simulink model "EnvironmentalControlSystem"  (R2018b)
settings: Solver=FixedStepAuto  StartTime=0.0  StopTime=500  FixedStep=0.01  RelTol=1e-3
values from neighbouring files (symbols this model uses):
  dt = 0.01    [run_sim.m]    (also in sys_id_pipeline.m = mean(diff(Time_vec_full)))
  K31 = Result31.K_slope    [sys_id_pipeline.m]
  K32 = Result32.K_slope    [sys_id_pipeline.m]
  P_ref = GlobalParams.P_ref    [sys_id_pipeline.m]
  Patm = GlobalParams.Patm    [sys_id_pipeline.m]
  R_gas = GlobalParams.R    [sys_id_pipeline.m]
  T_ref = GlobalParams.T_ref    [sys_id_pipeline.m]
  Tau31 = 5    [sys_id_pipeline.m]
  Tau32 = 5    [sys_id_pipeline.m]
  Tp31 = Result31.Tp    [sys_id_pipeline.m]
  Tp32 = Result32.Tp    [sys_id_pipeline.m]
  V_vol = pi * (0.05)^2 * 5    (= 0.0392699081699)    [run_sim.m]
  X31_den = sys_X31.Denominator    [sys_id_value.m]
  X31_num = sys_X31.Numerator    [sys_id_value.m]
  X32_den = sys_X32.Denominator    [sys_id_value.m]
  X32_num = sys_X32.Numerator    [sys_id_value.m]
libraries: simulink x14
(part 1 of 3)
settings Model: Creator=ZhaoJiance  LastModifiedBy=ZhaoJiance

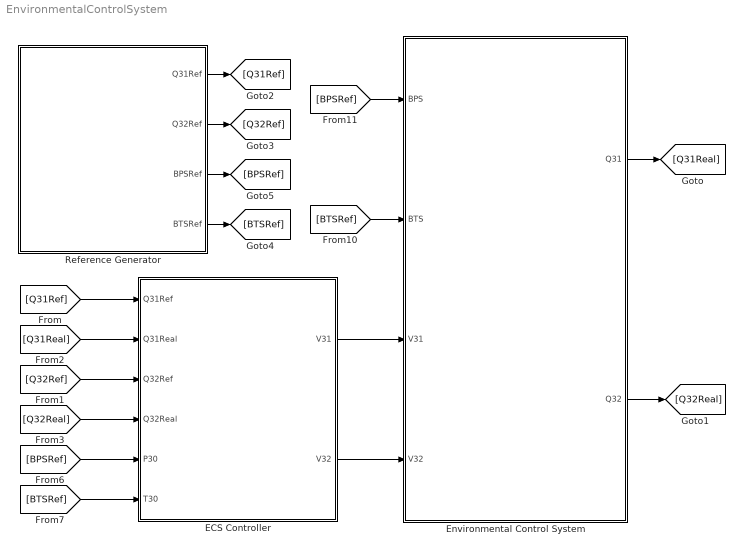
== system EnvironmentalControlSystem ==
  ECS Controller : Subsystem  VariantControlMode=Label  Variant=on  VariantControl=Variant1  LabelModeActiveChoice=Smith_MPC_Controller
  Environmental Control System : Subsystem
  Reference Generator : Subsystem
  wires:
  Reference Generator/4(BTSRef) -> [BTSRef]
  Reference Generator/2(Q32Ref) -> [Q32Ref]
  Reference Generator/3(BPSRef) -> [BPSRef]
  [BPSRef] -> Environmental Control System/1(BPS)
  [Q31Real] -> ECS Controller/2("Q31Real ")
  [BTSRef] -> Environmental Control System/2(BTS)
  [BTSRef] -> ECS Controller/6("T30 ")
  [Q32Ref] -> ECS Controller/3("Q32Ref ")
  [BPSRef] -> ECS Controller/5("P30 ")
  [Q31Ref] -> ECS Controller/1("Q31Ref ")
  Reference Generator/1(Q31Ref) -> [Q31Ref]
  [Q32Real] -> ECS Controller/4("Q32Real ")
  ECS Controller/1(" V31") -> Environmental Control System/3(V31)
  Environmental Control System/1(Q31) -> [Q31Real]
  ECS Controller/2(" V32") -> Environmental Control System/4(V32)
  Environmental Control System/2(Q32) -> [Q32Real]

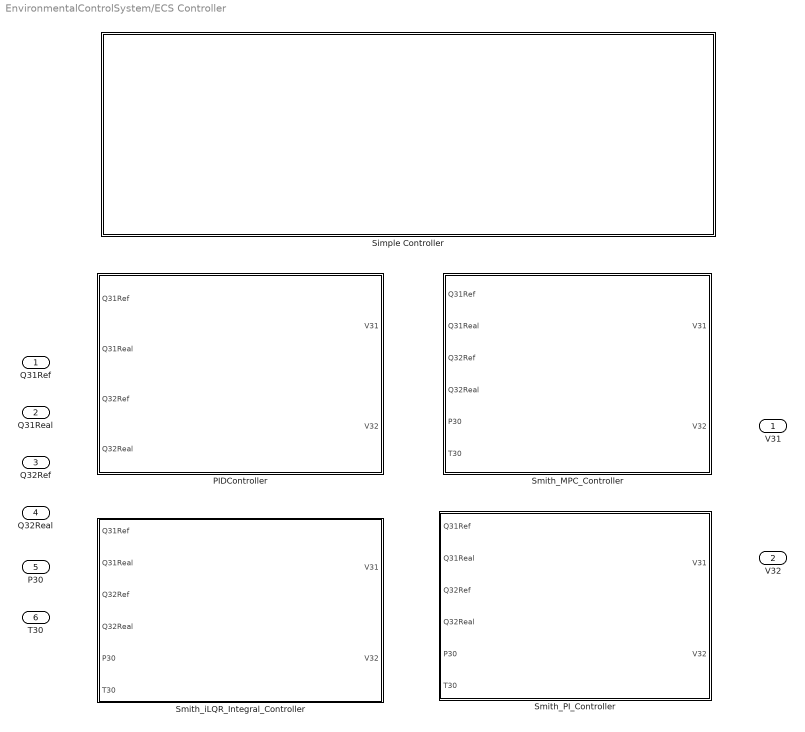
== system EnvironmentalControlSystem/ECS Controller ==
  "Q31Ref " : Inport
  "Q31Real " : Inport  Port=2
  "Q32Ref " : Inport  Port=3
  "Q32Real " : Inport  Port=4
  "P30 " : Inport  Port=5
  "T30 " : Inport  Port=6
  PIDController : Subsystem  VariantControl=PID
  Simple Controller : Subsystem  VariantControl=Variant
  Smith_MPC_Controller : Subsystem  VariantControl=Smith_MPC_Controller
  Smith_PI_Controller : Subsystem  VariantControl=Smith_PI_Controller
  Smith_iLQR_Integral_Controller : Subsystem  VariantControl=Smith_iLQR_Integral_Controller
  " V31" : Outport
  " V32" : Outport  Port=2

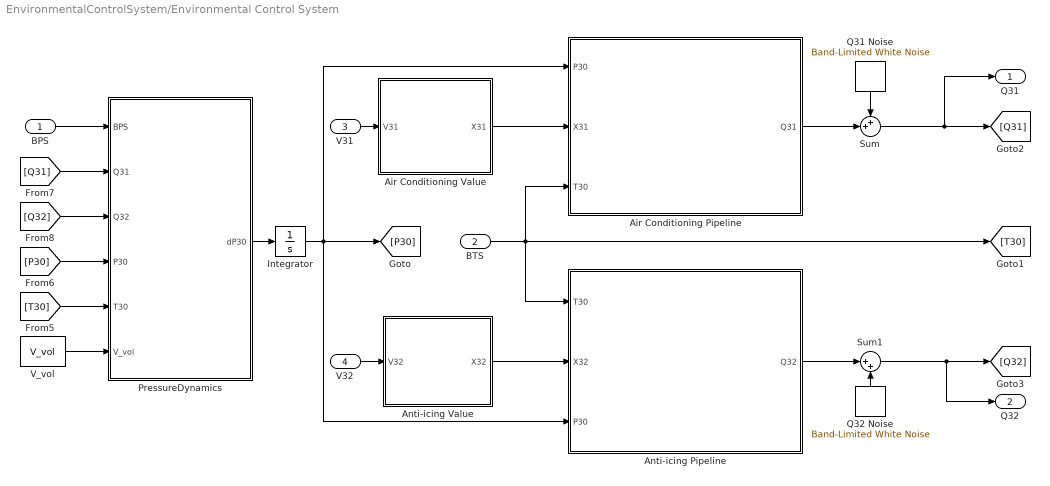
== system EnvironmentalControlSystem/Environmental Control System ==
  BPS : Inport
  BTS : Inport  Port=2
  V31 : Inport  Port=3
  V32 : Inport  Port=4
  Air Conditioning Pipeline : Subsystem
  Air Conditioning Value : Subsystem
  "Anti-icing Pipeline " : Subsystem
  Anti-icing Value : Subsystem
  Integrator : Integrator
  PressureDynamics : MATLAB Function  TreatAsAtomicUnit=on
  Q31 Noise : simulink/Sources/Band-Limited White Noise  Cov=Knoise  Ts=0.01  seed=[23341]
  Q32 Noise : simulink/Sources/Band-Limited White Noise  Cov=Knoise  Ts=0.01  seed=[23341]
  Sum : Sum  Inputs=++|
  Sum1 : Sum  Inputs=|++
  V_vol : Constant  Value=V_vol
  Q31 : Outport
  Q32 : Outport  Port=2
  wires:
  Air Conditioning Value/1(X31) -> Air Conditioning Pipeline/2(X31)
  BPS/1 -> PressureDynamics/1(BPS)
  Integrator/1 -> "Anti-icing Pipeline "/3(P30), [P30], Air Conditioning Pipeline/1(P30)
  Anti-icing Value/1(X32) -> "Anti-icing Pipeline "/2(X32)
  V31/1 -> Air Conditioning Value/1(V31)
  PressureDynamics/1(dP30) -> Integrator/1
  [Q32] -> PressureDynamics/3(Q32)
  [Q31] -> PressureDynamics/2(Q31)
  V_vol/1 -> PressureDynamics/6(V_vol)
  [P30] -> PressureDynamics/4(P30)
  [T30] -> PressureDynamics/5(T30)
  BTS/1 -> Air Conditioning Pipeline/3(T30), [T30], "Anti-icing Pipeline "/1(T30)
  Sum/1 -> [Q31], Q31/1
  Sum1/1 -> Q32/1, [Q32]
  Q32 Noise/1 -> Sum1/2
  "Anti-icing Pipeline "/1(Q32) -> Sum1/1
  Air Conditioning Pipeline/1(Q31) -> Sum/2
  Q31 Noise/1 -> Sum/1
  V32/1 -> Anti-icing Value/1(V32)

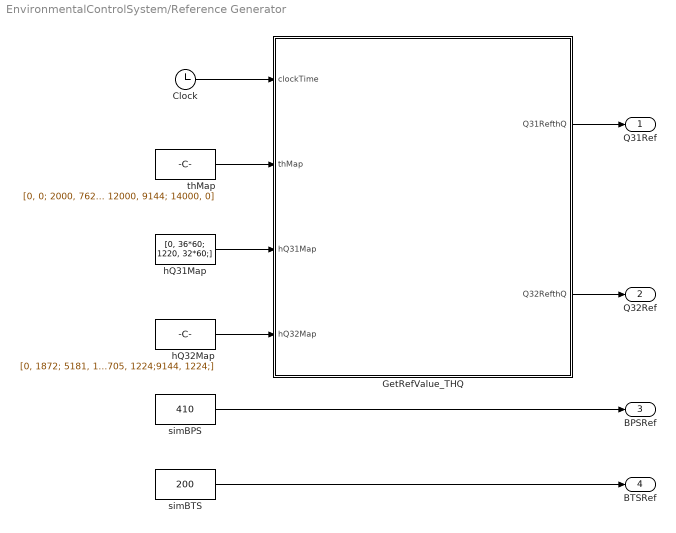
== system EnvironmentalControlSystem/Reference Generator ==
  Clock : Clock
  GetRefValue_THQ : MATLAB Function  TreatAsAtomicUnit=on
  hQ31Map : Constant  Value=[0, 36*60; 1220, 32*60;]
  hQ32Map : Constant  Value=[0, 1872; 5181, 1872; 6705, 1224;9144, 1224;]
  simBPS : Constant  Value=410
  simBTS : Constant  Value=200
  thMap : Constant  Value=[0, 0; 2000, 7620; 4000, 7620;6000, 12192; 8000, 12192; 10000, 9144; 12000, 9144; 14000, 0]
  Q31Ref : Outport
  Q32Ref : Outport  Port=2
  BPSRef : Outport  Port=3
  BTSRef : Outport  Port=4
  wires:
  Clock/1 -> GetRefValue_THQ/1(clockTime)
  thMap/1 -> GetRefValue_THQ/2(thMap)
  hQ31Map/1 -> GetRefValue_THQ/3(hQ31Map)
  hQ32Map/1 -> GetRefValue_THQ/4(hQ32Map)
  simBTS/1 -> BTSRef/1
  simBPS/1 -> BPSRef/1
  GetRefValue_THQ/1(Q31RefthQ) -> Q31Ref/1
  GetRefValue_THQ/2(Q32RefthQ) -> Q32Ref/1

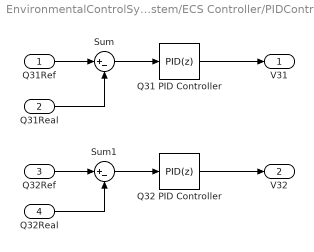
== system EnvironmentalControlSystem/ECS Controller/PIDController ==
  Q31Ref : Inport
  Q31Real : Inport  Port=2
  Q32Ref : Inport  Port=3
  Q32Real : Inport  Port=4
  Q31 PID Controller : simulink/Continuous/PID Controller  Controller=PID  Form=Parallel  TimeDomain=Discrete-time  SampleTime=-1  IntegratorMethod=Forward Euler  FilterMethod=Forward Euler  ControllerParametersSource=internal  P=0.0332634866006577  I=0.00162963841502539  D=0.0693776015925971  UseFilter=on  N=0.140831158638555  TunerSelectOption=Transfer Function Based (PID Tuner App)  InitialConditionSource=internal  InitialConditionForIntegrator=0  InitialConditionForFilter=0  DifferentiatorICPrevScaledInput=0  ExternalReset=none  TrackingMode=off  Kt=1  LimitOutput=off  UpperSaturationLimit=inf  LowerSaturationLimit=-inf  LinearizeAsGain=on  AntiWindupMode=none  Kb=1  POutMin=[]  POutMax=[]  IOutMin=[]  IOutMax=[]  DOutMin=[]  DOutMax=[]  NOutMin=[]  NOutMax=[]  SumOutMin=[]  SumOutMax=[]  SaturationOutMin=[]  SaturationOutMax=[]  PParamMin=[]  PParamMax=[]  IParamMin=[]  IParamMax=[]  DParamMin=[]  DParamMax=[]  NParamMin=[]  NParamMax=[]  KbParamMin=[]  KbParamMax=[]  KtParamMin=[]  KtParamMax=[]  KbOutMin=[]  KbOutMax=[]  KtOutMin=[]  KtOutMax=[]  IntegratorOutMin=[]  IntegratorOutMax=[]  FilterOutMin=[]  FilterOutMax=[]  SumI1OutMin=[]  SumI1OutMax=[]  SumI2OutMin=[]  SumI2OutMax=[]  SumI3OutMin=[]  SumI3OutMax=[]  SumI4OutMin=[]  SumI4OutMax=[]  SumDOutMin=[]  SumDOutMax=[]  DifferentiatorOutMin=[]  DifferentiatorOutMax=[]  FilterDiffOutCoefMin=[]  FilterDiffOutCoefMax=[]  ReciprocalOutMin=[]  ReciprocalOutMax=[]  SumDenOutMin=[]  SumDenOutMax=[]  SumNumOutMin=[]  SumNumOutMax=[]  DivideOutMin=[]  DivideOutMax=[]  IntegratorContinuousStateAttributes=''  IntegratorStateMustResolveToSignalObject=off  IntegratorRTWStateStorageClass=Auto  FilterContinuousStateAttributes=''  FilterStateMustResolveToSignalObject=off  FilterRTWStateStorageClass=Auto  ParallelPVariant=InternalParameters  IdealPVariant=Disabled  IVariant=InternalParameters  DVariant=InternalParameters  IntegratorVariant=Discrete  SatVariant=Disabled  AWVariant=Passthrough  PCopyVariant=Disabled  TRVariant=Disabled  FdbkBlocksVariant=Forward  IdealPFdbkVariant=Disabled  SatFdbkVariant=Disabled  DerivativeFilterVariant=ForwardEulerFilter  NVariant=InternalParameters  NCopyVariant=Disabled  FilterICVariant=InternalICsFilter  IntegratorICVariant=InternalICs  ExternalResetVariant=Disabled  TRSumVariant=Passthrough  SumFdbkVariant=Disabled  SumVariant=Sum_PID
  Q32 PID Controller : simulink/Continuous/PID Controller  Controller=PID  Form=Parallel  TimeDomain=Discrete-time  SampleTime=-1  IntegratorMethod=Forward Euler  FilterMethod=Forward Euler  ControllerParametersSource=internal  P=0.0550164924963942  I=0.00248684748202474  D=0.0884119468512251  UseFilter=on  N=14.1148734165854  TunerSelectOption=Transfer Function Based (PID Tuner App)  InitialConditionSource=internal  InitialConditionForIntegrator=0  InitialConditionForFilter=0  DifferentiatorICPrevScaledInput=0  ExternalReset=none  TrackingMode=off  Kt=1  LimitOutput=off  UpperSaturationLimit=inf  LowerSaturationLimit=-inf  LinearizeAsGain=on  AntiWindupMode=none  Kb=1  POutMin=[]  POutMax=[]  IOutMin=[]  IOutMax=[]  DOutMin=[]  DOutMax=[]  NOutMin=[]  NOutMax=[]  SumOutMin=[]  SumOutMax=[]  SaturationOutMin=[]  SaturationOutMax=[]  PParamMin=[]  PParamMax=[]  IParamMin=[]  IParamMax=[]  DParamMin=[]  DParamMax=[]  NParamMin=[]  NParamMax=[]  KbParamMin=[]  KbParamMax=[]  KtParamMin=[]  KtParamMax=[]  KbOutMin=[]  KbOutMax=[]  KtOutMin=[]  KtOutMax=[]  IntegratorOutMin=[]  IntegratorOutMax=[]  FilterOutMin=[]  FilterOutMax=[]  SumI1OutMin=[]  SumI1OutMax=[]  SumI2OutMin=[]  SumI2OutMax=[]  SumI3OutMin=[]  SumI3OutMax=[]  SumI4OutMin=[]  SumI4OutMax=[]  SumDOutMin=[]  SumDOutMax=[]  DifferentiatorOutMin=[]  DifferentiatorOutMax=[]  FilterDiffOutCoefMin=[]  FilterDiffOutCoefMax=[]  ReciprocalOutMin=[]  ReciprocalOutMax=[]  SumDenOutMin=[]  SumDenOutMax=[]  SumNumOutMin=[]  SumNumOutMax=[]  DivideOutMin=[]  DivideOutMax=[]  IntegratorContinuousStateAttributes=''  IntegratorStateMustResolveToSignalObject=off  IntegratorRTWStateStorageClass=Auto  FilterContinuousStateAttributes=''  FilterStateMustResolveToSignalObject=off  FilterRTWStateStorageClass=Auto  ParallelPVariant=InternalParameters  IdealPVariant=Disabled  IVariant=InternalParameters  DVariant=InternalParameters  IntegratorVariant=Discrete  SatVariant=Disabled  AWVariant=Passthrough  PCopyVariant=Disabled  TRVariant=Disabled  FdbkBlocksVariant=Forward  IdealPFdbkVariant=Disabled  SatFdbkVariant=Disabled  DerivativeFilterVariant=ForwardEulerFilter  NVariant=InternalParameters  NCopyVariant=Disabled  FilterICVariant=InternalICsFilter  IntegratorICVariant=InternalICs  ExternalResetVariant=Disabled  TRSumVariant=Passthrough  SumFdbkVariant=Disabled  SumVariant=Sum_PID
  Sum : Sum  Inputs=|+-
  Sum1 : Sum  Inputs=|+-
  V31 : Outport
  V32 : Outport  Port=2
  wires:
  Q31Ref/1 -> Sum/1
  Sum/1 -> Q31 PID Controller/1
  Q32Real/1 -> Sum1/2
  Q32Ref/1 -> Sum1/1
  Q31Real/1 -> Sum/2
  Q31 PID Controller/1 -> V31/1
  Q32 PID Controller/1 -> V32/1
  Sum1/1 -> Q32 PID Controller/1

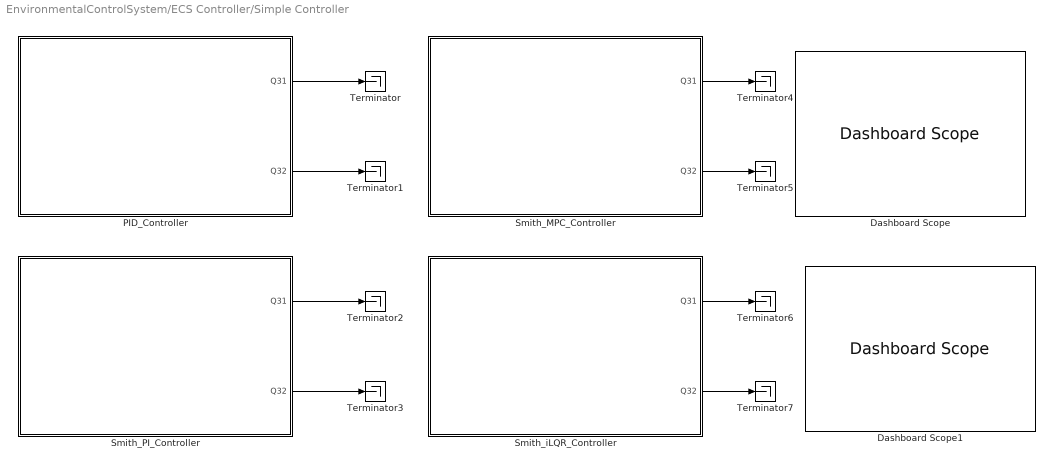
== system EnvironmentalControlSystem/ECS Controller/Simple Controller ==
  Dashboard Scope : DashboardScope  WebBlockId=462
  Dashboard Scope1 : DashboardScope  WebBlockId=463
  PID_Controller : Subsystem
  Smith_MPC_Controller : Subsystem
  Smith_PI_Controller : Subsystem
  Smith_iLQR_Controller : Subsystem
  Terminator{,1..7} (8 alike) : Terminator
  wires:
  Smith_iLQR_Controller/1(Q31) -> Terminator6/1
  PID_Controller/1(Q31) -> Terminator/1
  Smith_iLQR_Controller/2(Q32) -> Terminator7/1
  Smith_PI_Controller/2(Q32) -> Terminator3/1
  Smith_MPC_Controller/1(Q31) -> Terminator4/1
  PID_Controller/2(Q32) -> Terminator1/1
  Smith_MPC_Controller/2(Q32) -> Terminator5/1
  Smith_PI_Controller/1(Q31) -> Terminator2/1

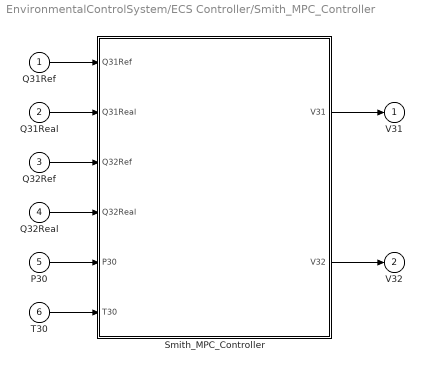
== system EnvironmentalControlSystem/ECS Controller/Smith_MPC_Controller ==
  "Q31Ref " : Inport
  "Q31Real " : Inport  Port=2
  "Q32Ref " : Inport  Port=3
  "Q32Real " : Inport  Port=4
  "P30 " : Inport  Port=5
  "T30 " : Inport  Port=6
  Smith_MPC_Controller : MATLAB Function  TreatAsAtomicUnit=on
  " V31" : Outport
  " V32" : Outport  Port=2
  wires:
  "Q31Ref "/1 -> Smith_MPC_Controller/1(Q31Ref)
  "Q31Real "/1 -> Smith_MPC_Controller/2(Q31Real)
  "T30 "/1 -> Smith_MPC_Controller/6(T30)
  "P30 "/1 -> Smith_MPC_Controller/5(P30)
  "Q32Real "/1 -> Smith_MPC_Controller/4(Q32Real)
  "Q32Ref "/1 -> Smith_MPC_Controller/3(Q32Ref)
  Smith_MPC_Controller/2(V32) -> " V32"/1
  Smith_MPC_Controller/1(V31) -> " V31"/1

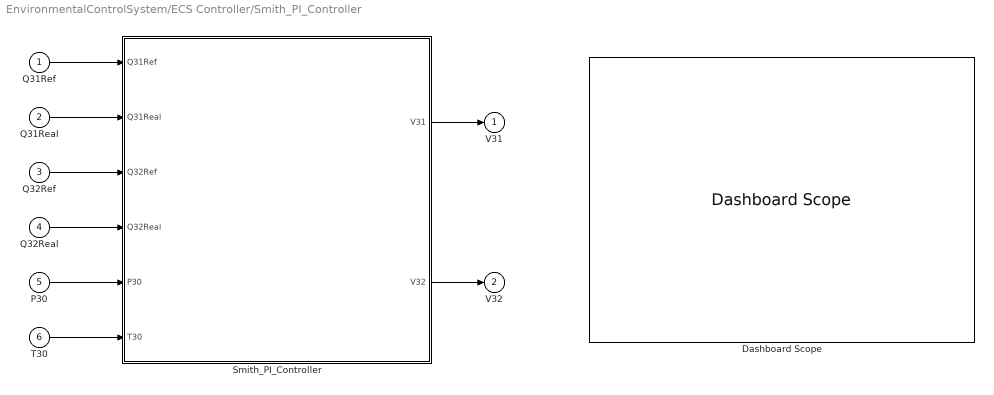
== system EnvironmentalControlSystem/ECS Controller/Smith_PI_Controller ==
  "Q31Ref " : Inport
  "Q31Real " : Inport  Port=2
  "Q32Ref " : Inport  Port=3
  "Q32Real " : Inport  Port=4
  "P30 " : Inport  Port=5
  "T30 " : Inport  Port=6
  Dashboard Scope : DashboardScope  WebBlockId=445
  Smith_PI_Controller : MATLAB Function  TreatAsAtomicUnit=on
  " V31" : Outport
  " V32" : Outport  Port=2
  wires:
  Smith_PI_Controller/1(V31) -> " V31"/1
  Smith_PI_Controller/2(V32) -> " V32"/1
  "Q31Ref "/1 -> Smith_PI_Controller/1(Q31Ref)
  "Q31Real "/1 -> Smith_PI_Controller/2(Q31Real)
  "Q32Ref "/1 -> Smith_PI_Controller/3(Q32Ref)
  "Q32Real "/1 -> Smith_PI_Controller/4(Q32Real)
  "P30 "/1 -> Smith_PI_Controller/5(P30)
  "T30 "/1 -> Smith_PI_Controller/6(T30)

== system EnvironmentalControlSystem/ECS Controller/Smith_iLQR_Integral_Controller ==
  "Q31Ref " : Inport
  "Q31Real " : Inport  Port=2
  "Q32Ref " : Inport  Port=3
  "Q32Real " : Inport  Port=4
  "P30 " : Inport  Port=5
  "T30 " : Inport  Port=6
  Smith_iLQR_Integral_Controller : MATLAB Function  TreatAsAtomicUnit=on
  " V31" : Outport
  " V32" : Outport  Port=2
  wires:
  Smith_iLQR_Integral_Controller/1(V31) -> " V31"/1
  Smith_iLQR_Integral_Controller/2(V32) -> " V32"/1
  "Q31Real "/1 -> Smith_iLQR_Integral_Controller/2(Q31Real)
  "Q31Ref "/1 -> Smith_iLQR_Integral_Controller/1(Q31Ref)
  "Q32Ref "/1 -> Smith_iLQR_Integral_Controller/3(Q32Ref)
  "Q32Real "/1 -> Smith_iLQR_Integral_Controller/4(Q32Real)
  "P30 "/1 -> Smith_iLQR_Integral_Controller/5(P30)
  "T30 "/1 -> Smith_iLQR_Integral_Controller/6(T30)

== system EnvironmentalControlSystem/Environmental Control System/Air Conditioning Pipeline ==
  P30 : Inport
  X31 : Inport  Port=2
  T30 : Inport  Port=3
  MATLAB Function : MATLAB Function  TreatAsAtomicUnit=on
  Saturation : Saturate  UpperLimit=inf  LowerLimit=0
  Transfer Fcn : TransferFcn  Denominator=[Tp31 1]
  Transport Delay : TransportDelay  DelayTime=Tau31
  Q31 : Outport
  wires:
  Transfer Fcn/1 -> Transport Delay/1
  X31/1 -> MATLAB Function/1(X)
  MATLAB Function/1(Q_static) -> Transfer Fcn/1
  T30/1 -> MATLAB Function/3(T30)
  P30/1 -> MATLAB Function/2(P30)
  Transport Delay/1 -> Saturation/1
  Saturation/1 -> Q31/1

== system EnvironmentalControlSystem/Environmental Control System/Air Conditioning Value ==
  V31 : Inport
  V31Saturation : Saturate  UpperLimit=100  LowerLimit=0
  X31 Saturation : Saturate  UpperLimit=100  LowerLimit=0
  X31 Value System : TransferFcn  Numerator=X31_num  Denominator=X31_den
  X31Deadband : MATLAB Function  TreatAsAtomicUnit=on  SystemSampleTime=0.01
  X31 : Outport
  wires:
  X31Deadband/1(u_eff) -> X31 Value System/1
  X31 Saturation/1 -> X31/1, X31Deadband/1(curPos)
  X31 Value System/1 -> X31 Saturation/1
  V31/1 -> V31Saturation/1
  V31Saturation/1 -> X31Deadband/2(cmdPos)

== system EnvironmentalControlSystem/Environmental Control System/Anti-icing Pipeline  ==
  T30 : Inport
  X32 : Inport  Port=2
  P30 : Inport  Port=3
  MATLAB Function : MATLAB Function  TreatAsAtomicUnit=on
  Saturation : Saturate  UpperLimit=inf  LowerLimit=0
  Transfer Fcn : TransferFcn  Denominator=[Tp32 1]
  Transport Delay : TransportDelay  DelayTime=Tau32
  Q32 : Outport
  wires:
  P30/1 -> MATLAB Function/2(P30)
  MATLAB Function/1(Q_static) -> Transfer Fcn/1
  Transfer Fcn/1 -> Transport Delay/1
  T30/1 -> MATLAB Function/3(T30)
  Transport Delay/1 -> Saturation/1
  X32/1 -> MATLAB Function/1(X)
  Saturation/1 -> Q32/1

== system EnvironmentalControlSystem/Environmental Control System/Anti-icing Value ==
  V32 : Inport
  V32 Saturation : Saturate  UpperLimit=100  LowerLimit=0
  X32 Saturation : Saturate  UpperLimit=100  LowerLimit=0
  X32 Value System : TransferFcn  Numerator=X32_num  Denominator=X32_den
  X32Deadband : MATLAB Function  TreatAsAtomicUnit=on  SystemSampleTime=0.01
  X32 : Outport
  wires:
  V32/1 -> V32 Saturation/1
  X32Deadband/1(u_eff) -> X32 Value System/1
  X32 Saturation/1 -> X32/1, X32Deadband/1(curPos)
  X32 Value System/1 -> X32 Saturation/1
  V32 Saturation/1 -> X32Deadband/2(cmdPos)

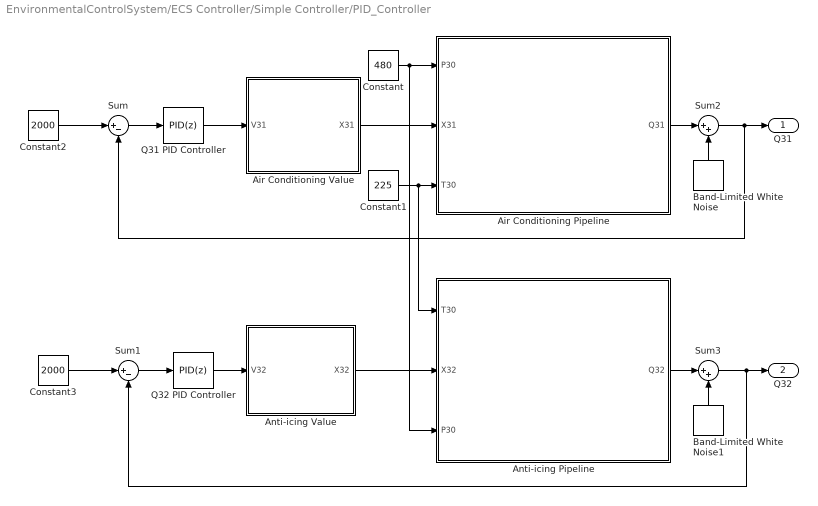
== system EnvironmentalControlSystem/ECS Controller/Simple Controller/PID_Controller ==
  Air Conditioning Pipeline : Subsystem
  Air Conditioning Value : Subsystem
  "Anti-icing Pipeline " : Subsystem
  Anti-icing Value : Subsystem
  Band-Limited White Noise : simulink/Sources/Band-Limited White Noise  Cov=Knoise  Ts=0.1  seed=[23341]
  Band-Limited White Noise1 : simulink/Sources/Band-Limited White Noise  Cov=Knoise  Ts=0.1  seed=[23341]
  Constant : Constant  Value=480
  Constant1 : Constant  Value=225
  Constant2 : Constant  Value=2000
  Constant3 : Constant  Value=2000
  Q31 PID Controller : simulink/Continuous/PID Controller  Controller=PID  Form=Parallel  TimeDomain=Discrete-time  SampleTime=-1  IntegratorMethod=Forward Euler  FilterMethod=Forward Euler  ControllerParametersSource=internal  P=0.0332634866006577  I=0.00162963841502539  D=0.0693776015925971  UseFilter=on  N=0.140831158638555  TunerSelectOption=Transfer Function Based (PID Tuner App)  InitialConditionSource=internal  InitialConditionForIntegrator=0  InitialConditionForFilter=0  DifferentiatorICPrevScaledInput=0  ExternalReset=none  TrackingMode=off  Kt=1  LimitOutput=off  UpperSaturationLimit=inf  LowerSaturationLimit=-inf  LinearizeAsGain=on  AntiWindupMode=none  Kb=1  POutMin=[]  POutMax=[]  IOutMin=[]  IOutMax=[]  DOutMin=[]  DOutMax=[]  NOutMin=[]  NOutMax=[]  SumOutMin=[]  SumOutMax=[]  SaturationOutMin=[]  SaturationOutMax=[]  PParamMin=[]  PParamMax=[]  IParamMin=[]  IParamMax=[]  DParamMin=[]  DParamMax=[]  NParamMin=[]  NParamMax=[]  KbParamMin=[]  KbParamMax=[]  KtParamMin=[]  KtParamMax=[]  KbOutMin=[]  KbOutMax=[]  KtOutMin=[]  KtOutMax=[]  IntegratorOutMin=[]  IntegratorOutMax=[]  FilterOutMin=[]  FilterOutMax=[]  SumI1OutMin=[]  SumI1OutMax=[]  SumI2OutMin=[]  SumI2OutMax=[]  SumI3OutMin=[]  SumI3OutMax=[]  SumI4OutMin=[]  SumI4OutMax=[]  SumDOutMin=[]  SumDOutMax=[]  DifferentiatorOutMin=[]  DifferentiatorOutMax=[]  FilterDiffOutCoefMin=[]  FilterDiffOutCoefMax=[]  ReciprocalOutMin=[]  ReciprocalOutMax=[]  SumDenOutMin=[]  SumDenOutMax=[]  SumNumOutMin=[]  SumNumOutMax=[]  DivideOutMin=[]  DivideOutMax=[]  IntegratorContinuousStateAttributes=''  IntegratorStateMustResolveToSignalObject=off  IntegratorRTWStateStorageClass=Auto  FilterContinuousStateAttributes=''  FilterStateMustResolveToSignalObject=off  FilterRTWStateStorageClass=Auto  ParallelPVariant=InternalParameters  IdealPVariant=Disabled  IVariant=InternalParameters  DVariant=InternalParameters  IntegratorVariant=Discrete  SatVariant=Disabled  AWVariant=Passthrough  PCopyVariant=Disabled  TRVariant=Disabled  FdbkBlocksVariant=Forward  IdealPFdbkVariant=Disabled  SatFdbkVariant=Disabled  DerivativeFilterVariant=ForwardEulerFilter  NVariant=InternalParameters  NCopyVariant=Disabled  FilterICVariant=InternalICsFilter  IntegratorICVariant=InternalICs  ExternalResetVariant=Disabled  TRSumVariant=Passthrough  SumFdbkVariant=Disabled  SumVariant=Sum_PID
  Q32 PID Controller : simulink/Continuous/PID Controller  Controller=PID  Form=Parallel  TimeDomain=Discrete-time  SampleTime=-1  IntegratorMethod=Forward Euler  FilterMethod=Forward Euler  ControllerParametersSource=internal  P=0.0550164924963942  I=0.00248684748202474  D=0.0884119468512251  UseFilter=on  N=14.1148734165854  TunerSelectOption=Transfer Function Based (PID Tuner App)  InitialConditionSource=internal  InitialConditionForIntegrator=0  InitialConditionForFilter=0  DifferentiatorICPrevScaledInput=0  ExternalReset=none  TrackingMode=off  Kt=1  LimitOutput=off  UpperSaturationLimit=inf  LowerSaturationLimit=-inf  LinearizeAsGain=on  AntiWindupMode=none  Kb=1  POutMin=[]  POutMax=[]  IOutMin=[]  IOutMax=[]  DOutMin=[]  DOutMax=[]  NOutMin=[]  NOutMax=[]  SumOutMin=[]  SumOutMax=[]  SaturationOutMin=[]  SaturationOutMax=[]  PParamMin=[]  PParamMax=[]  IParamMin=[]  IParamMax=[]  DParamMin=[]  DParamMax=[]  NParamMin=[]  NParamMax=[]  KbParamMin=[]  KbParamMax=[]  KtParamMin=[]  KtParamMax=[]  KbOutMin=[]  KbOutMax=[]  KtOutMin=[]  KtOutMax=[]  IntegratorOutMin=[]  IntegratorOutMax=[]  FilterOutMin=[]  FilterOutMax=[]  SumI1OutMin=[]  SumI1OutMax=[]  SumI2OutMin=[]  SumI2OutMax=[]  SumI3OutMin=[]  SumI3OutMax=[]  SumI4OutMin=[]  SumI4OutMax=[]  SumDOutMin=[]  SumDOutMax=[]  DifferentiatorOutMin=[]  DifferentiatorOutMax=[]  FilterDiffOutCoefMin=[]  FilterDiffOutCoefMax=[]  ReciprocalOutMin=[]  ReciprocalOutMax=[]  SumDenOutMin=[]  SumDenOutMax=[]  SumNumOutMin=[]  SumNumOutMax=[]  DivideOutMin=[]  DivideOutMax=[]  IntegratorContinuousStateAttributes=''  IntegratorStateMustResolveToSignalObject=off  IntegratorRTWStateStorageClass=Auto  FilterContinuousStateAttributes=''  FilterStateMustResolveToSignalObject=off  FilterRTWStateStorageClass=Auto  ParallelPVariant=InternalParameters  IdealPVariant=Disabled  IVariant=InternalParameters  DVariant=InternalParameters  IntegratorVariant=Discrete  SatVariant=Disabled  AWVariant=Passthrough  PCopyVariant=Disabled  TRVariant=Disabled  FdbkBlocksVariant=Forward  IdealPFdbkVariant=Disabled  SatFdbkVariant=Disabled  DerivativeFilterVariant=ForwardEulerFilter  NVariant=InternalParameters  NCopyVariant=Disabled  FilterICVariant=InternalICsFilter  IntegratorICVariant=InternalICs  ExternalResetVariant=Disabled  TRSumVariant=Passthrough  SumFdbkVariant=Disabled  SumVariant=Sum_PID
  Sum : Sum  Inputs=|+-
  Sum1 : Sum  Inputs=|+-
  Sum2 : Sum  Inputs=|++
  Sum3 : Sum  Inputs=|++
  Q31 : Outport
  Q32 : Outport  Port=2
  wires:
  Sum1/1 -> Q32 PID Controller/1
  Constant/1 -> Air Conditioning Pipeline/1(P30), "Anti-icing Pipeline "/3(P30)
  Anti-icing Value/1(X32) -> "Anti-icing Pipeline "/2(X32)
  Sum/1 -> Q31 PID Controller/1
  Constant3/1 -> Sum1/1
  Constant2/1 -> Sum/1
  Q31 PID Controller/1 -> Air Conditioning Value/1(V31)
  Constant1/1 -> "Anti-icing Pipeline "/1(T30), Air Conditioning Pipeline/3(T30)
  Air Conditioning Value/1(X31) -> Air Conditioning Pipeline/2(X31)
  Q32 PID Controller/1 -> Anti-icing Value/1(V32)
  Band-Limited White Noise1/1 -> Sum3/2
  Sum3/1 -> Q32/1, Sum1/2
  Band-Limited White Noise/1 -> Sum2/2
  Air Conditioning Pipeline/1(Q31) -> Sum2/1
  Sum2/1 -> Sum/2, Q31/1
  "Anti-icing Pipeline "/1(Q32) -> Sum3/1

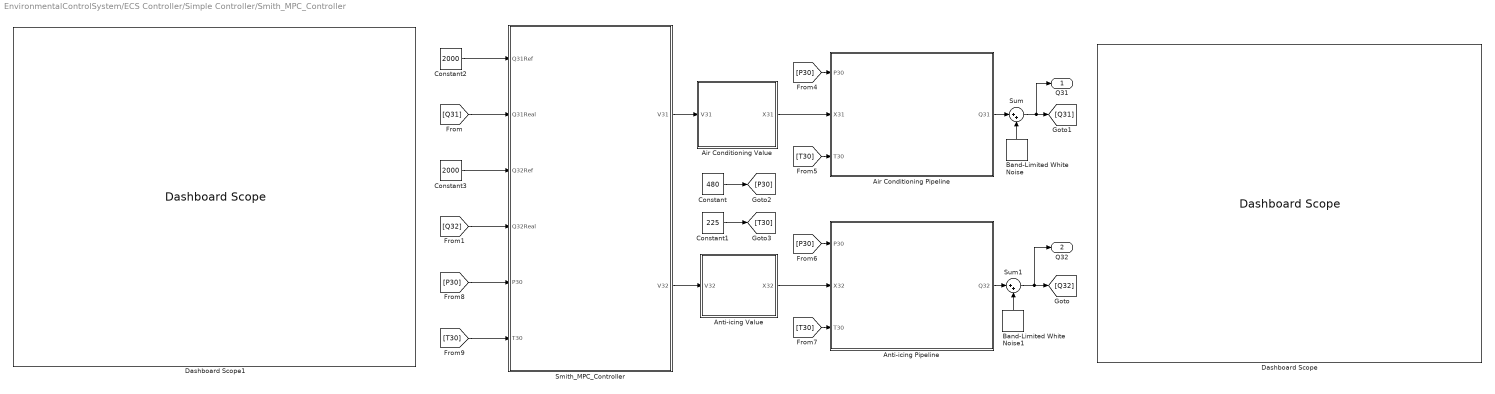
== system EnvironmentalControlSystem/ECS Controller/Simple Controller/Smith_MPC_Controller ==
  Air Conditioning Pipeline : Subsystem
  Air Conditioning Value : Subsystem
  "Anti-icing Pipeline " : Subsystem
  Anti-icing Value : Subsystem
  Band-Limited White Noise : simulink/Sources/Band-Limited White Noise  Cov=Knoise  Ts=0.1  seed=[23341]
  Band-Limited White Noise1 : simulink/Sources/Band-Limited White Noise  Cov=Knoise  Ts=0.1  seed=[23341]
  Constant : Constant  Value=480
  Constant1 : Constant  Value=225
  Constant2 : Constant  Value=2000
  Constant3 : Constant  Value=2000
  Dashboard Scope : DashboardScope  WebBlockId=550
  Dashboard Scope1 : DashboardScope  WebBlockId=551
  Smith_MPC_Controller : MATLAB Function  TreatAsAtomicUnit=on
  Sum : Sum  Inputs=|++
  Sum1 : Sum  Inputs=|++
  Q31 : Outport
  Q32 : Outport  Port=2
  wires:
  Anti-icing Value/1(X32) -> "Anti-icing Pipeline "/2(X32)
  Smith_MPC_Controller/1(V31) -> Air Conditioning Value/1(V31)
  Air Conditioning Value/1(X31) -> Air Conditioning Pipeline/2(X31)
  Constant2/1 -> Smith_MPC_Controller/1(Q31Ref)
  Band-Limited White Noise/1 -> Sum/2
  Air Conditioning Pipeline/1(Q31) -> Sum/1
  Sum/1 -> [Q31], Q31/1
  Band-Limited White Noise1/1 -> Sum1/2
  "Anti-icing Pipeline "/1(Q32) -> Sum1/1
  Sum1/1 -> [Q32], Q32/1
  Smith_MPC_Controller/2(V32) -> Anti-icing Value/1(V32)
  [Q31] -> Smith_MPC_Controller/2(Q31Real)
  [P30] -> Air Conditioning Pipeline/1(P30)
  [T30] -> Air Conditioning Pipeline/3(T30)
  [T30] -> "Anti-icing Pipeline "/3(T30)
  [P30] -> "Anti-icing Pipeline "/1(P30)
  Constant/1 -> [P30]
  Constant1/1 -> [T30]
  [T30] -> Smith_MPC_Controller/6(T30)
  Constant3/1 -> Smith_MPC_Controller/3(Q32Ref)
  [P30] -> Smith_MPC_Controller/5(P30)
  [Q32] -> Smith_MPC_Controller/4(Q32Real)

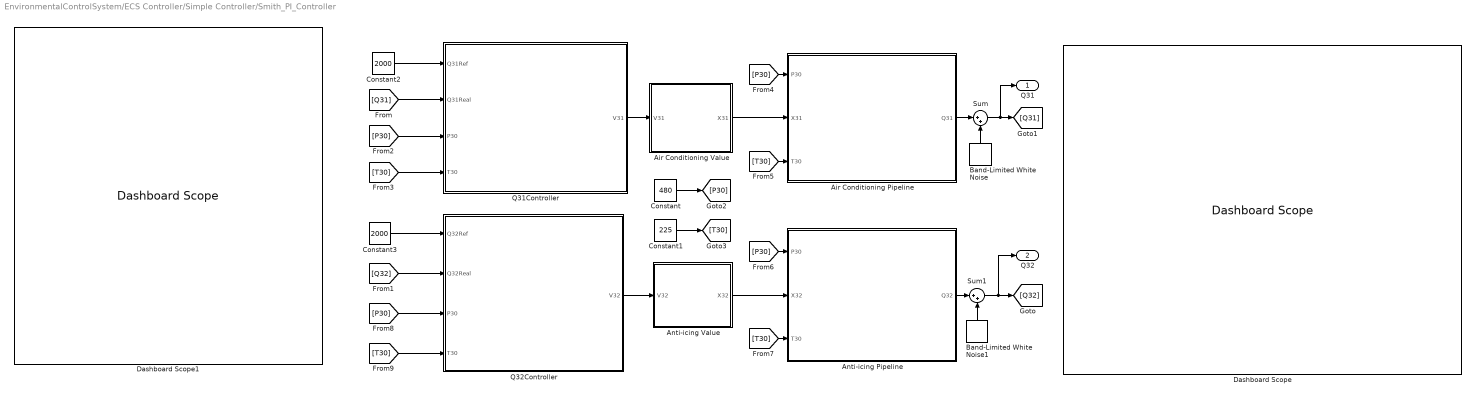
== system EnvironmentalControlSystem/ECS Controller/Simple Controller/Smith_PI_Controller ==
  Air Conditioning Pipeline : Subsystem
  Air Conditioning Value : Subsystem
  "Anti-icing Pipeline " : Subsystem
  Anti-icing Value : Subsystem
  Band-Limited White Noise : simulink/Sources/Band-Limited White Noise  Cov=Knoise  Ts=0.1  seed=[23341]
  Band-Limited White Noise1 : simulink/Sources/Band-Limited White Noise  Cov=Knoise  Ts=0.1  seed=[23341]
  Constant : Constant  Value=480
  Constant1 : Constant  Value=225
  Constant2 : Constant  Value=2000
  Constant3 : Constant  Value=2000
  Dashboard Scope : DashboardScope  WebBlockId=608
  Dashboard Scope1 : DashboardScope  WebBlockId=609
  Q31Controller : MATLAB Function  TreatAsAtomicUnit=on
  Q32Controller : MATLAB Function  TreatAsAtomicUnit=on
  Sum : Sum  Inputs=|++
  Sum1 : Sum  Inputs=|++
  Q31 : Outport
  Q32 : Outport  Port=2
  wires:
  [P30] -> Q31Controller/3(P30)
  Anti-icing Value/1(X32) -> "Anti-icing Pipeline "/2(X32)
  Q31Controller/1(V31) -> Air Conditioning Value/1(V31)
  Air Conditioning Value/1(X31) -> Air Conditioning Pipeline/2(X31)
  Constant2/1 -> Q31Controller/1(Q31Ref)
  [T30] -> Q31Controller/4(T30)
  Band-Limited White Noise/1 -> Sum/2
  Air Conditioning Pipeline/1(Q31) -> Sum/1
  Sum/1 -> [Q31], Q31/1
  Band-Limited White Noise1/1 -> Sum1/2
  "Anti-icing Pipeline "/1(Q32) -> Sum1/1
  Sum1/1 -> [Q32], Q32/1
  Q32Controller/1(V32) -> Anti-icing Value/1(V32)
  [Q31] -> Q31Controller/2(Q31Real)
  [P30] -> Air Conditioning Pipeline/1(P30)
  [T30] -> Air Conditioning Pipeline/3(T30)
  [T30] -> "Anti-icing Pipeline "/3(T30)
  [P30] -> "Anti-icing Pipeline "/1(P30)
  Constant/1 -> [P30]
  Constant1/1 -> [T30]
  [Q32] -> Q32Controller/2(Q32Real)
  [T30] -> Q32Controller/4(T30)
  Constant3/1 -> Q32Controller/1(Q32Ref)
  [P30] -> Q32Controller/3(P30)

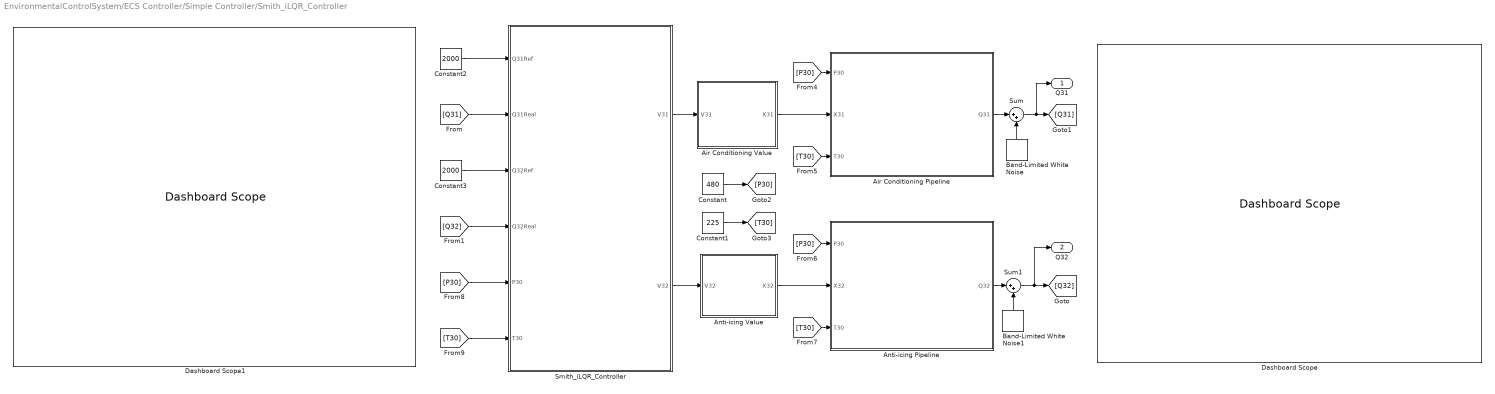
== system EnvironmentalControlSystem/ECS Controller/Simple Controller/Smith_iLQR_Controller ==
  Air Conditioning Pipeline : Subsystem
  Air Conditioning Value : Subsystem
  "Anti-icing Pipeline " : Subsystem
  Anti-icing Value : Subsystem
  Band-Limited White Noise : simulink/Sources/Band-Limited White Noise  Cov=Knoise  Ts=0.1  seed=[23341]
  Band-Limited White Noise1 : simulink/Sources/Band-Limited White Noise  Cov=Knoise  Ts=0.1  seed=[23341]
  Constant : Constant  Value=480
  Constant1 : Constant  Value=225
  Constant2 : Constant  Value=2000
  Constant3 : Constant  Value=2000
  Dashboard Scope : DashboardScope  WebBlockId=669
  Dashboard Scope1 : DashboardScope  WebBlockId=670
  Smith_iLQR_Controller : MATLAB Function  TreatAsAtomicUnit=on
  Sum : Sum  Inputs=|++
  Sum1 : Sum  Inputs=|++
  Q31 : Outport
  Q32 : Outport  Port=2
  wires:
  Anti-icing Value/1(X32) -> "Anti-icing Pipeline "/2(X32)
  Smith_iLQR_Controller/1(V31) -> Air Conditioning Value/1(V31)
  Air Conditioning Value/1(X31) -> Air Conditioning Pipeline/2(X31)
  Constant2/1 -> Smith_iLQR_Controller/1(Q31Ref)
  Band-Limited White Noise/1 -> Sum/2
  Air Conditioning Pipeline/1(Q31) -> Sum/1
  Sum/1 -> [Q31], Q31/1
  Band-Limited White Noise1/1 -> Sum1/2
  "Anti-icing Pipeline "/1(Q32) -> Sum1/1
  Sum1/1 -> [Q32], Q32/1
  Smith_iLQR_Controller/2(V32) -> Anti-icing Value/1(V32)
  [Q31] -> Smith_iLQR_Controller/2(Q31Real)
  [P30] -> Air Conditioning Pipeline/1(P30)
  [T30] -> Air Conditioning Pipeline/3(T30)
  [T30] -> "Anti-icing Pipeline "/3(T30)
  [P30] -> "Anti-icing Pipeline "/1(P30)
  Constant/1 -> [P30]
  Constant1/1 -> [T30]
  [T30] -> Smith_iLQR_Controller/6(T30)
  Constant3/1 -> Smith_iLQR_Controller/3(Q32Ref)
  [P30] -> Smith_iLQR_Controller/5(P30)
  [Q32] -> Smith_iLQR_Controller/4(Q32Real)

== system EnvironmentalControlSystem/ECS Controller/Simple Controller/PID_Controller/Air Conditioning Pipeline ==
  P30 : Inport
  X31 : Inport  Port=2
  T30 : Inport  Port=3
  MATLAB Function : MATLAB Function  TreatAsAtomicUnit=on
  Saturation : Saturate  UpperLimit=inf  LowerLimit=0
  Transfer Fcn : TransferFcn  Denominator=[Tp31 1]
  Transport Delay : TransportDelay  DelayTime=Tau31
  Q31 : Outport
  wires:
  Transfer Fcn/1 -> Transport Delay/1
  X31/1 -> MATLAB Function/1(X)
  MATLAB Function/1(Q_static) -> Transfer Fcn/1
  T30/1 -> MATLAB Function/3(T30)
  P30/1 -> MATLAB Function/2(P30)
  Transport Delay/1 -> Saturation/1
  Saturation/1 -> Q31/1

== system EnvironmentalControlSystem/ECS Controller/Simple Controller/PID_Controller/Air Conditioning Value ==
  V31 : Inport
  V31Saturation : Saturate  UpperLimit=100  LowerLimit=0
  X31 Saturation : Saturate  UpperLimit=100  LowerLimit=0
  X31 Value System : TransferFcn  Numerator=X31_num  Denominator=X31_den
  X31Deadband : MATLAB Function  TreatAsAtomicUnit=on  SystemSampleTime=0.01
  X31 : Outport
  wires:
  X31Deadband/1(u_eff) -> X31 Value System/1
  X31 Saturation/1 -> X31/1, X31Deadband/1(curPos)
  X31 Value System/1 -> X31 Saturation/1
  V31/1 -> V31Saturation/1
  V31Saturation/1 -> X31Deadband/2(cmdPos)

== system EnvironmentalControlSystem/ECS Controller/Simple Controller/PID_Controller/Anti-icing Pipeline  ==
  T30 : Inport
  X32 : Inport  Port=2
  P30 : Inport  Port=3
  MATLAB Function : MATLAB Function  TreatAsAtomicUnit=on
  Saturation : Saturate  UpperLimit=inf  LowerLimit=0
  Transfer Fcn : TransferFcn  Denominator=[Tp32 1]
  Transport Delay : TransportDelay  DelayTime=Tau32
  Q32 : Outport
  wires:
  P30/1 -> MATLAB Function/2(P30)
  MATLAB Function/1(Q_static) -> Transfer Fcn/1
  Transfer Fcn/1 -> Transport Delay/1
  T30/1 -> MATLAB Function/3(T30)
  Transport Delay/1 -> Saturation/1
  X32/1 -> MATLAB Function/1(X)
  Saturation/1 -> Q32/1

== system EnvironmentalControlSystem/ECS Controller/Simple Controller/PID_Controller/Anti-icing Value ==
  V32 : Inport
  V32 Saturation : Saturate  UpperLimit=100  LowerLimit=0
  X32 Saturation : Saturate  UpperLimit=100  LowerLimit=0
  X32 Value System : TransferFcn  Numerator=X32_num  Denominator=X32_den
  X32Deadband : MATLAB Function  TreatAsAtomicUnit=on  SystemSampleTime=0.01
  X32 : Outport
  wires:
  V32/1 -> V32 Saturation/1
  X32Deadband/1(u_eff) -> X32 Value System/1
  X32 Saturation/1 -> X32/1, X32Deadband/1(curPos)
  X32 Value System/1 -> X32 Saturation/1
  V32 Saturation/1 -> X32Deadband/2(cmdPos)

== system EnvironmentalControlSystem/ECS Controller/Simple Controller/Smith_MPC_Controller/Air Conditioning Pipeline ==
  P30 : Inport
  X31 : Inport  Port=2
  T30 : Inport  Port=3
  MATLAB Function : MATLAB Function  TreatAsAtomicUnit=on
  Saturation : Saturate  UpperLimit=inf  LowerLimit=0
  Transfer Fcn : TransferFcn  Denominator=[Tp31 1]
  Transport Delay : TransportDelay  DelayTime=Tau31
  Q31 : Outport
  wires:
  Transfer Fcn/1 -> Transport Delay/1
  X31/1 -> MATLAB Function/1(X)
  MATLAB Function/1(Q_static) -> Transfer Fcn/1
  T30/1 -> MATLAB Function/3(T30)
  P30/1 -> MATLAB Function/2(P30)
  Transport Delay/1 -> Saturation/1
  Saturation/1 -> Q31/1

== system EnvironmentalControlSystem/ECS Controller/Simple Controller/Smith_MPC_Controller/Air Conditioning Value ==
  V31 : Inport
  V31Saturation : Saturate  UpperLimit=100  LowerLimit=0
  X31 Saturation : Saturate  UpperLimit=100  LowerLimit=0
  X31 Value System : TransferFcn  Numerator=X31_num  Denominator=X31_den
  X31Deadband : MATLAB Function  TreatAsAtomicUnit=on  SystemSampleTime=0.01
  X31 : Outport
  wires:
  X31Deadband/1(u_eff) -> X31 Value System/1
  X31 Saturation/1 -> X31/1, X31Deadband/1(curPos)
  X31 Value System/1 -> X31 Saturation/1
  V31/1 -> V31Saturation/1
  V31Saturation/1 -> X31Deadband/2(cmdPos)

== system EnvironmentalControlSystem/ECS Controller/Simple Controller/Smith_MPC_Controller/Anti-icing Pipeline  ==
  P30 : Inport
  X32 : Inport  Port=2
  T30 : Inport  Port=3
  MATLAB Function : MATLAB Function  TreatAsAtomicUnit=on
  Saturation : Saturate  UpperLimit=inf  LowerLimit=0
  Transfer Fcn : TransferFcn  Denominator=[Tp32 1]
  Transport Delay : TransportDelay  DelayTime=Tau32
  Q32 : Outport
  wires:
  P30/1 -> MATLAB Function/2(P30)
  MATLAB Function/1(Q_static) -> Transfer Fcn/1
  Transfer Fcn/1 -> Transport Delay/1
  T30/1 -> MATLAB Function/3(T30)
  Transport Delay/1 -> Saturation/1
  X32/1 -> MATLAB Function/1(X)
  Saturation/1 -> Q32/1

== system EnvironmentalControlSystem/ECS Controller/Simple Controller/Smith_MPC_Controller/Anti-icing Value ==
  V32 : Inport
  V32 Saturation : Saturate  UpperLimit=100  LowerLimit=0
  X32 Saturation : Saturate  UpperLimit=100  LowerLimit=0
  X32 Value System : TransferFcn  Numerator=X32_num  Denominator=X32_den
  X32Deadband : MATLAB Function  TreatAsAtomicUnit=on  SystemSampleTime=0.01
  X32 : Outport
  wires:
  V32/1 -> V32 Saturation/1
  X32Deadband/1(u_eff) -> X32 Value System/1
  X32 Saturation/1 -> X32/1, X32Deadband/1(curPos)
  X32 Value System/1 -> X32 Saturation/1
  V32 Saturation/1 -> X32Deadband/2(cmdPos)

== system EnvironmentalControlSystem/ECS Controller/Simple Controller/Smith_PI_Controller/Air Conditioning Pipeline ==
  P30 : Inport
  X31 : Inport  Port=2
  T30 : Inport  Port=3
  MATLAB Function : MATLAB Function  TreatAsAtomicUnit=on
  Saturation : Saturate  UpperLimit=inf  LowerLimit=0
  Transfer Fcn : TransferFcn  Denominator=[Tp31 1]
  Transport Delay : TransportDelay  DelayTime=Tau31
  Q31 : Outport
  wires:
  Transfer Fcn/1 -> Transport Delay/1
  X31/1 -> MATLAB Function/1(X)
  MATLAB Function/1(Q_static) -> Transfer Fcn/1
  T30/1 -> MATLAB Function/3(T30)
  P30/1 -> MATLAB Function/2(P30)
  Transport Delay/1 -> Saturation/1
  Saturation/1 -> Q31/1

== system EnvironmentalControlSystem/ECS Controller/Simple Controller/Smith_PI_Controller/Air Conditioning Value ==
  V31 : Inport
  V31Saturation : Saturate  UpperLimit=100  LowerLimit=0
  X31 Saturation : Saturate  UpperLimit=100  LowerLimit=0
  X31 Value System : TransferFcn  Numerator=X31_num  Denominator=X31_den
  X31Deadband : MATLAB Function  TreatAsAtomicUnit=on  SystemSampleTime=0.01
  X31 : Outport
  wires:
  X31Deadband/1(u_eff) -> X31 Value System/1
  X31 Saturation/1 -> X31/1, X31Deadband/1(curPos)
  X31 Value System/1 -> X31 Saturation/1
  V31/1 -> V31Saturation/1
  V31Saturation/1 -> X31Deadband/2(cmdPos)

== system EnvironmentalControlSystem/ECS Controller/Simple Controller/Smith_PI_Controller/Anti-icing Pipeline  ==
  P30 : Inport
  X32 : Inport  Port=2
  T30 : Inport  Port=3
  MATLAB Function : MATLAB Function  TreatAsAtomicUnit=on
  Saturation : Saturate  UpperLimit=inf  LowerLimit=0
  Transfer Fcn : TransferFcn  Denominator=[Tp32 1]
  Transport Delay : TransportDelay  DelayTime=Tau32
  Q32 : Outport
  wires:
  P30/1 -> MATLAB Function/2(P30)
  MATLAB Function/1(Q_static) -> Transfer Fcn/1
  Transfer Fcn/1 -> Transport Delay/1
  T30/1 -> MATLAB Function/3(T30)
  Transport Delay/1 -> Saturation/1
  X32/1 -> MATLAB Function/1(X)
  Saturation/1 -> Q32/1

== system EnvironmentalControlSystem/ECS Controller/Simple Controller/Smith_PI_Controller/Anti-icing Value ==
  V32 : Inport
  V32 Saturation : Saturate  UpperLimit=100  LowerLimit=0
  X32 Saturation : Saturate  UpperLimit=100  LowerLimit=0
  X32 Value System : TransferFcn  Numerator=X32_num  Denominator=X32_den
  X32Deadband : MATLAB Function  TreatAsAtomicUnit=on  SystemSampleTime=0.01
  X32 : Outport
  wires:
  V32/1 -> V32 Saturation/1
  X32Deadband/1(u_eff) -> X32 Value System/1
  X32 Saturation/1 -> X32/1, X32Deadband/1(curPos)
  X32 Value System/1 -> X32 Saturation/1
  V32 Saturation/1 -> X32Deadband/2(cmdPos)

== system EnvironmentalControlSystem/ECS Controller/Simple Controller/Smith_iLQR_Controller/Air Conditioning Pipeline ==
  P30 : Inport
  X31 : Inport  Port=2
  T30 : Inport  Port=3
  MATLAB Function : MATLAB Function  TreatAsAtomicUnit=on
  Saturation : Saturate  UpperLimit=inf  LowerLimit=0
  Transfer Fcn : TransferFcn  Denominator=[Tp31 1]
  Transport Delay : TransportDelay  DelayTime=Tau31
  Q31 : Outport
  wires:
  Transfer Fcn/1 -> Transport Delay/1
  X31/1 -> MATLAB Function/1(X)
  MATLAB Function/1(Q_static) -> Transfer Fcn/1
  T30/1 -> MATLAB Function/3(T30)
  P30/1 -> MATLAB Function/2(P30)
  Transport Delay/1 -> Saturation/1
  Saturation/1 -> Q31/1

== system EnvironmentalControlSystem/ECS Controller/Simple Controller/Smith_iLQR_Controller/Air Conditioning Value ==
  V31 : Inport
  V31Saturation : Saturate  UpperLimit=100  LowerLimit=0
  X31 Saturation : Saturate  UpperLimit=100  LowerLimit=0
  X31 Value System : TransferFcn  Numerator=X31_num  Denominator=X31_den
  X31Deadband : MATLAB Function  TreatAsAtomicUnit=on  SystemSampleTime=0.01
  X31 : Outport
  wires:
  X31Deadband/1(u_eff) -> X31 Value System/1
  X31 Saturation/1 -> X31/1, X31Deadband/1(curPos)
  X31 Value System/1 -> X31 Saturation/1
  V31/1 -> V31Saturation/1
  V31Saturation/1 -> X31Deadband/2(cmdPos)

== system EnvironmentalControlSystem/ECS Controller/Simple Controller/Smith_iLQR_Controller/Anti-icing Pipeline  ==
  P30 : Inport
  X32 : Inport  Port=2
  T30 : Inport  Port=3
  MATLAB Function : MATLAB Function  TreatAsAtomicUnit=on
  Saturation : Saturate  UpperLimit=inf  LowerLimit=0
  Transfer Fcn : TransferFcn  Denominator=[Tp32 1]
  Transport Delay : TransportDelay  DelayTime=Tau32
  Q32 : Outport
  wires:
  P30/1 -> MATLAB Function/2(P30)
  MATLAB Function/1(Q_static) -> Transfer Fcn/1
  Transfer Fcn/1 -> Transport Delay/1
  T30/1 -> MATLAB Function/3(T30)
  Transport Delay/1 -> Saturation/1
  X32/1 -> MATLAB Function/1(X)
  Saturation/1 -> Q32/1

== system EnvironmentalControlSystem/ECS Controller/Simple Controller/Smith_iLQR_Controller/Anti-icing Value ==
  V32 : Inport
  V32 Saturation : Saturate  UpperLimit=100  LowerLimit=0
  X32 Saturation : Saturate  UpperLimit=100  LowerLimit=0
  X32 Value System : TransferFcn  Numerator=X32_num  Denominator=X32_den
  X32Deadband : MATLAB Function  TreatAsAtomicUnit=on  SystemSampleTime=0.01
  X32 : Outport
  wires:
  V32/1 -> V32 Saturation/1
  X32Deadband/1(u_eff) -> X32 Value System/1
  X32 Saturation/1 -> X32/1, X32Deadband/1(curPos)
  X32 Value System/1 -> X32 Saturation/1
  V32 Saturation/1 -> X32Deadband/2(cmdPos)

== matlab function EnvironmentalControlSystem/Environmental Control System/Anti-icing Value/X32Deadband ==
  data: curPos input; u_eff output; cmdPos input
function u_eff = X32Deadband(curPos, cmdPos)
    % 引入持久变量来记录系统当前的状态：是在"调节中"还是"已到位"
    persistent isAdjusting
    if isempty(isAdjusting)
        isAdjusting = false;
    end

    % === 参数设置 ===
    % Start_Deadband: 启动死区（防抖阈值）。误差超过此值，开始动作
    % 设为 3，意味着噪声在 +/-3 以内时，若系统本来是静止的，就不理会
    Start_Deadband = 2.0; 
    
    % Stop_Deadband: 停止死区（精度阈值）。误差小于此值，才算到位
    % 设为 0.5，意味着一旦动起来，必须修到 99.5~100.5 之间才停手
    Stop_Deadband  = 0.2; 

    % 计算当前误差绝对值
    err = abs(cmdPos - curPos);

    % === 状态机逻辑 ===
    if isAdjusting
        % 【状态1：正在调节中】
        % 既然已经动起来了，就要追求高精度。
        % 只有当误差足够小（满足精度要求）时，才停止。
        if err <= Stop_Deadband
            isAdjusting = false; % 切换状态：认为已到位
            u_eff = curPos;      % 欺骗控制器误差为0，使其停止积分/输出
        else
            isAdjusting = true;  % 保持调节状态
            u_eff = cmdPos;      % 正常输出目标值给控制器
        end
    else
        % 【状态2：已到位/静止中】
        % 此时为了防抖，对小误差视而不见。
        % 只有当误差突然变大（超过启动阈值，比如新指令来了）时，才开始动
        if err > Start_Deadband
            isAdjusting = true;  % 切换状态：开始调节
            u_eff = cmdPos;      % 输出目标值
        else
            isAdjusting = false; % 保持静止
            u_eff = curPos;      % 锁定当前位置，抑制抖动
        end
    end
end

== matlab function EnvironmentalControlSystem/Environmental Control System/Air Conditioning Value/X31Deadband ==
  data: curPos input; u_eff output; cmdPos input
function u_eff = X31Deadband(curPos, cmdPos)
    % 引入持久变量来记录系统当前的状态：是在"调节中"还是"已到位"
    persistent isAdjusting
    if isempty(isAdjusting)
        isAdjusting = false;
    end

    % === 参数设置 ===
    % Start_Deadband: 启动死区（防抖阈值）。误差超过此值，开始动作
    % 设为 3，意味着噪声在 +/-3 以内时，若系统本来是静止的，就不理会
    Start_Deadband = 2.0; 
    
    % Stop_Deadband: 停止死区（精度阈值）。误差小于此值，才算到位
    % 设为 0.5，意味着一旦动起来，必须修到 99.5~100.5 之间才停手
    Stop_Deadband  = 0.2; 

    % 计算当前误差绝对值
    err = abs(cmdPos - curPos);

    % === 状态机逻辑 ===
    if isAdjusting
        % 【状态1：正在调节中】
        % 既然已经动起来了，就要追求高精度。
        % 只有当误差足够小（满足精度要求）时，才停止。
        if err <= Stop_Deadband
            isAdjusting = false; % 切换状态：认为已到位
            u_eff = curPos;      % 欺骗控制器误差为0，使其停止积分/输出
        else
            isAdjusting = true;  % 保持调节状态
            u_eff = cmdPos;      % 正常输出目标值给控制器
        end
    else
        % 【状态2：已到位/静止中】
        % 此时为了防抖，对小误差视而不见。
        % 只有当误差突然变大（超过启动阈值，比如新指令来了）时，才开始动
        if err > Start_Deadband
            isAdjusting = true;  % 切换状态：开始调节
            u_eff = cmdPos;      % 输出目标值
        else
            isAdjusting = false; % 保持静止
            u_eff = curPos;      % 锁定当前位置，抑制抖动
        end
    end
end

== matlab function EnvironmentalControlSystem/Environmental Control System/Air Conditioning Pipeline/MATLAB Function ==
  data: X input; Q_static output; P30 input; T30 input; K31 parameter; P_ref parameter; T_ref parameter; R_gas parameter; Patm parameter
function Q_static = StaticCalc(X, P30, T30, K31, P_ref, T_ref, R_gas, Patm)
    % 输入单位说明:
    % X: 阀门开度 (0-1 或 0-100，取决于你的K是基于什么单位)
    % P_dyn: 实时压力 (kPa)
    % T_dyn: 实时温度 (摄氏度)
    
    % --- 1. 计算标称流量 (Nominal Flow) ---
    Q_nominal = K31 * X;
    
    % --- 2. 计算实时物理因子 (Real-time Term) ---
    % 温度转开尔文
    Tk_dyn = T30 + 273.15;
    delta_P_dyn = P30 - Patm;
    Term_Dyn = sqrt(max((P30 * delta_P_dyn) / (R_gas * Tk_dyn), 0));
    
    % --- 3. 计算参考物理因子 (Reference Term - Constant) ---
    Tk_ref = T_ref + 273.15;
    delta_P_ref = P_ref - Patm;
    Term_Ref = sqrt(max((P_ref * delta_P_ref) / (R_gas * Tk_ref), 0));
    
    % --- 4. 计算最终静态流量 (修正后) ---
    if Term_Ref < 1e-6
        Ratio = 1;
    else
        Ratio = Term_Dyn / Term_Ref;
    end
    
    Q_static = Q_nominal * Ratio;
end

== matlab function EnvironmentalControlSystem/Environmental Control System/Anti-icing Pipeline /MATLAB Function ==
  data: X input; Q_static output; P30 input; T30 input; K32 parameter; P_ref parameter; T_ref parameter; R_gas parameter; Patm parameter
function Q_static = StaticCalc(X, P30, T30, K32, P_ref, T_ref, R_gas, Patm)
    % 输入单位说明:
    % X: 阀门开度 (0-1 或 0-100，取决于你的K是基于什么单位)
    % P_dyn: 实时压力 (kPa)
    % T_dyn: 实时温度 (摄氏度)
    
    % --- 1. 计算标称流量 (Nominal Flow) ---
    Q_nominal = K32 * X;
    
    % --- 2. 计算实时物理因子 (Real-time Term) ---
    % 温度转开尔文
    Tk_dyn = T30 + 273.15;
    delta_P_dyn = P30 - Patm;
    Term_Dyn = sqrt(max((P30 * delta_P_dyn) / (R_gas * Tk_dyn), 0));
    
    % --- 3. 计算参考物理因子 (Reference Term - Constant) ---
    Tk_ref = T_ref + 273.15;
    delta_P_ref = P_ref - Patm;
    Term_Ref = sqrt(max((P_ref * delta_P_ref) / (R_gas * Tk_ref), 0));
    
    % --- 4. 计算最终静态流量 (修正后) ---
    if Term_Ref < 1e-6
        Ratio = 1;
    else
        Ratio = Term_Dyn / Term_Ref;
    end
    
    Q_static = Q_nominal * Ratio;
end

== matlab function EnvironmentalControlSystem/Environmental Control System/PressureDynamics ==
  data: BPS input; Q31 input; dP30 output; Q32 input; P30 input; T30 input; V_vol input; R_gas parameter
function dP30 = PressureDynamics(BPS, Q31, Q32, P30, T30, V_vol, R_gas)
    % 输入:
    % Q31, Q32: 两个支路的实时流量 (kg/h) -> 需转换为 kg/s
    % P30: 当前公共节点压力 (kPa) -> 需转换为 Pa
    % P_source: 气源总压力 (kPa)
    % V_vol: 管汇体积 (m^3)，这是一个调试参数，实际系统为2-4m长的DN100管路
    
    % --- 单位换算 ---
    Q_out_kgs = (Q31 + Q32) / 3600; % kg/h -> kg/s
    P30_Pa = P30 * 1000;
    P_source_Pa = BPS * 1000;
    T_K = T30 + 273.15;
    
    % --- 1. 计算气源供气流量 Q_in (模拟上游特性) ---
    % 假设上游是一个大减压阀或限流孔板，流量与压差有关
    % Kv_source 是上游供气能力的系数，需要大致估算
    Kv_source = 0.005; 
    
    if P_source_Pa > P30_Pa
        % 简化的亚音速/声速流动方程
        Q_in_kgs = Kv_source * sqrt(P_source_Pa - P30_Pa);
    else
        Q_in_kgs = 0;
    end
    
%     % 临界压力比 (空气 k=1.4)
%     Critical_Ratio = 0.528; % (2/(k+1))^(k/(k-1))
% 
%     if P30_Pa / P_source_Pa < Critical_Ratio
%         % --- 阻塞流 (Sonic / Choked) ---
%         % 流量主要取决于上游压力 BPS
%         % C_choked 是阻塞流系数，通常约为 Kv_source / sqrt(R*T) 的某种比例
%         Q_in_kgs = Kv_source * 0.5 * sqrt(P_source_Pa); % 这是一个简化的工程近似，需根据Kv定义调整
%     else
%         % --- 亚音速流 (Subsonic) ---
%         Q_in_kgs = Kv_source * sqrt(P_source_Pa - P30_Pa);
%     end
    
    % --- 2. 容腔微分方程 (dP/dt) ---
    % 根据理想气体状态方程微分形式: dP/dt = (RT/V) * (Qin - Qout)
    % 这是一个积分环节，体现了压力的建立过程
    
    dP_dt_Pa = (R_gas * T_K / V_vol) * (Q_in_kgs - Q_out_kgs);
    
    % --- 输出 ---
    dP30 = dP_dt_Pa / 1000; % 换回 kPa/s
end

== matlab function EnvironmentalControlSystem/ECS Controller/Simple Controller/Smith_MPC_Controller/Air Conditioning Pipeline/MATLAB Function ==
  data: X input; Q_static output; P30 input; T30 input; K31 parameter; P_ref parameter; T_ref parameter; R_gas parameter; Patm parameter
function Q_static = StaticCalc(X, P30, T30, K31, P_ref, T_ref, R_gas, Patm)
    % 输入单位说明:
    % X: 阀门开度 (0-1 或 0-100，取决于你的K是基于什么单位)
    % P_dyn: 实时压力 (kPa)
    % T_dyn: 实时温度 (摄氏度)
    
    % --- 1. 计算标称流量 (Nominal Flow) ---
    Q_nominal = K31 * X;
    
    % --- 2. 计算实时物理因子 (Real-time Term) ---
    % 温度转开尔文
    Tk_dyn = T30 + 273.15;
    delta_P_dyn = P30 - Patm;
    Term_Dyn = sqrt(max((P30 * delta_P_dyn) / (R_gas * Tk_dyn), 0));
    
    % --- 3. 计算参考物理因子 (Reference Term - Constant) ---
    Tk_ref = T_ref + 273.15;
    delta_P_ref = P_ref - Patm;
    Term_Ref = sqrt(max((P_ref * delta_P_ref) / (R_gas * Tk_ref), 0));
    
    % --- 4. 计算最终静态流量 (修正后) ---
    if Term_Ref < 1e-6
        Ratio = 1;
    else
        Ratio = Term_Dyn / Term_Ref;
    end
    
    Q_static = Q_nominal * Ratio;
end

== matlab function EnvironmentalControlSystem/ECS Controller/Simple Controller/Smith_MPC_Controller/Air Conditioning Value/X31Deadband ==
  data: curPos input; u_eff output; cmdPos input
function u_eff = X31Deadband(curPos, cmdPos)
    % 引入持久变量来记录系统当前的状态：是在"调节中"还是"已到位"
    persistent isAdjusting
    if isempty(isAdjusting)
        isAdjusting = false;
    end

    % === 参数设置 ===
    % Start_Deadband: 启动死区（防抖阈值）。误差超过此值，开始动作
    % 设为 3，意味着噪声在 +/-3 以内时，若系统本来是静止的，就不理会
    Start_Deadband = 2.0; 
    
    % Stop_Deadband: 停止死区（精度阈值）。误差小于此值，才算到位
    % 设为 0.5，意味着一旦动起来，必须修到 99.5~100.5 之间才停手
    Stop_Deadband  = 0.2; 

    % 计算当前误差绝对值
    err = abs(cmdPos - curPos);

    % === 状态机逻辑 ===
    if isAdjusting
        % 【状态1：正在调节中】
        % 既然已经动起来了，就要追求高精度。
        % 只有当误差足够小（满足精度要求）时，才停止。
        if err <= Stop_Deadband
            isAdjusting = false; % 切换状态：认为已到位
            u_eff = curPos;      % 欺骗控制器误差为0，使其停止积分/输出
        else
            isAdjusting = true;  % 保持调节状态
            u_eff = cmdPos;      % 正常输出目标值给控制器
        end
    else
        % 【状态2：已到位/静止中】
        % 此时为了防抖，对小误差视而不见。
        % 只有当误差突然变大（超过启动阈值，比如新指令来了）时，才开始动
        if err > Start_Deadband
            isAdjusting = true;  % 切换状态：开始调节
            u_eff = cmdPos;      % 输出目标值
        else
            isAdjusting = false; % 保持静止
            u_eff = curPos;      % 锁定当前位置，抑制抖动
        end
    end
end

== matlab function EnvironmentalControlSystem/ECS Controller/Simple Controller/Smith_MPC_Controller/Anti-icing Pipeline /MATLAB Function ==
  data: X input; Q_static output; P30 input; T30 input; K32 parameter; P_ref parameter; T_ref parameter; R_gas parameter; Patm parameter
function Q_static = StaticCalc(X, P30, T30, K32, P_ref, T_ref, R_gas, Patm)
    % 输入单位说明:
    % X: 阀门开度 (0-1 或 0-100，取决于你的K是基于什么单位)
    % P_dyn: 实时压力 (kPa)
    % T_dyn: 实时温度 (摄氏度)
    
    % --- 1. 计算标称流量 (Nominal Flow) ---
    Q_nominal = K32 * X;
    
    % --- 2. 计算实时物理因子 (Real-time Term) ---
    % 温度转开尔文
    Tk_dyn = T30 + 273.15;
    delta_P_dyn = P30 - Patm;
    Term_Dyn = sqrt(max((P30 * delta_P_dyn) / (R_gas * Tk_dyn), 0));
    
    % --- 3. 计算参考物理因子 (Reference Term - Constant) ---
    Tk_ref = T_ref + 273.15;
    delta_P_ref = P_ref - Patm;
    Term_Ref = sqrt(max((P_ref * delta_P_ref) / (R_gas * Tk_ref), 0));
    
    % --- 4. 计算最终静态流量 ---
    if Term_Ref < 1e-6
        Ratio = 1;
    else
        Ratio = Term_Dyn / Term_Ref;
    end
    
    Q_static = Q_nominal * Ratio;
end
